simulink model "cubesatAttSim"  (R2024a)
settings: Solver=FixedStepAuto  StartTime=0.0  StopTime=7200  FixedStep=0.02  MaxStep=1  MinStep=0.001  RelTol=1e-3
model workspace (MAT data in the model file):
  earth_magnetic_field_body = [0 0 0]
  initial_angular_momentum_body = 0
  initial_position_iss_orbit = 0
  initial_quaterion_rotation = 0
  initial_velocity_iss_orbit = 0
  intertia_tensor = 0
  mass = 0
  maximum_sun_sensor_vision = 0
  reference_magnetic_field_direction = 0
  reference_sun_direction = 0
  wheel_distribution_matrix = [1  0  0  0; 0  1  0  0; 0  0  1  1]
libraries: aerolibutil x2, sharedtransform x1
settings Model: Creator=samuel  LastModifiedBy=joshu
settings OptimizationCC: ReuseModelBlockBuffer=off
settings DebuggingCC: AlgebraicLoopMsg=error  ArtificialAlgebraicLoopMsg=error
settings ModelReferenceCC: EnableRefExpFcnMdlSchedulingChecks=on
settings RTWCC: GPUComputeCapability=3.5

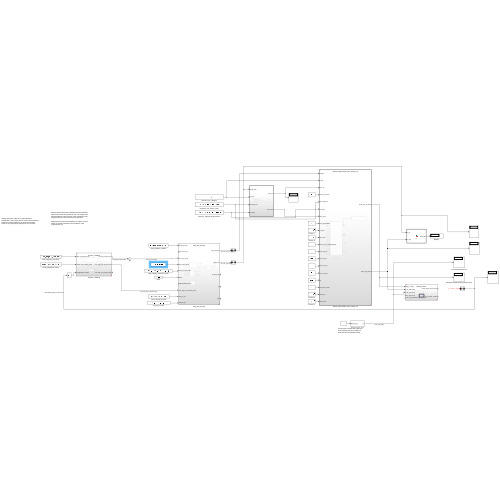
[thumbnail: Simulink's stored preview of the top-level diagram]
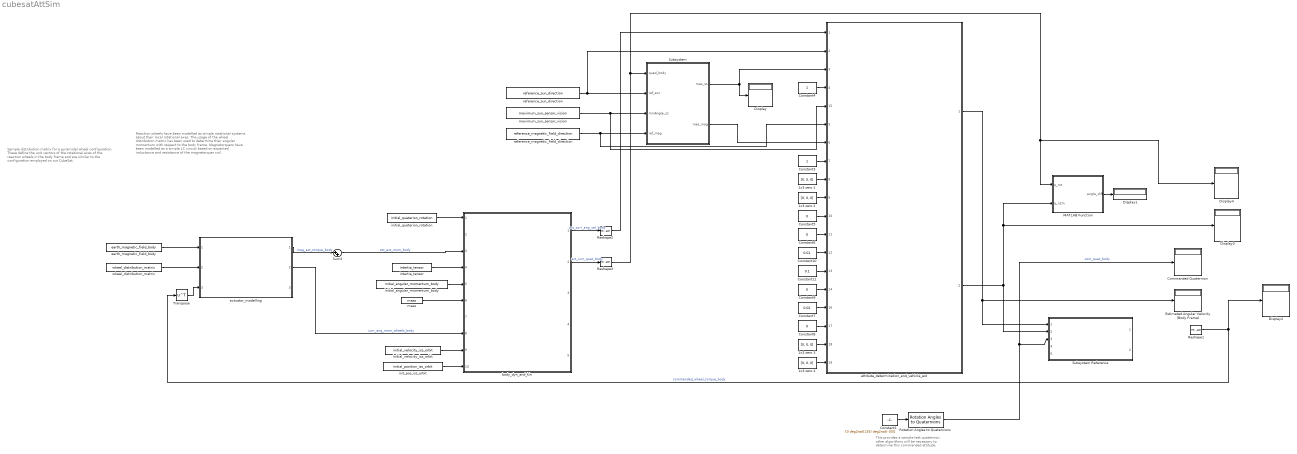
== system cubesatAttSim ==
  note: This provides a sample test quaternion, other algorithms will be necessary to determine this commanded attitude.
  note: Reaction wheels have been modelled as simple rotational systems about their local rotational axes. The usage of the wheel distribution matrix has been used to determine their angular momentum with respect to the body frame.
      |
      | Magnetorquers have been modelled as a simple LC circuit based on expected inductance and resistance of the magnetorquer coil.
  note: Sample distribution matrix for a pyramidal wheel configuration. These define the unit vectors of the rotational axes of the reaction wheels in the body frame and are similar to the configuration employed on our CubeSat.
  1x3 zero {1..4} (4 alike) : Constant  Value=[0, 0, 0]
  Commanded Quaternion : Display
  Constant1 : Constant  Value=[0 deg2rad(135) deg2rad(-30)]
  Constant10 : Constant  Value=0.01
  Constant11 : Constant  Value=0.1
  Constant3 : Constant  OutDataTypeStr=boolean
  Constant4 : Constant  OutDataTypeStr=boolean
  Constant5 : Constant  Value=0  OutDataTypeStr=boolean
  Constant6 : Constant  Value=0  OutDataTypeStr=boolean
  Constant7 : Constant  Value=0.02
  Constant8 : Constant  Value=0  OutDataTypeStr=boolean
  Constant9 : Constant  Value=0
  Display{,1..4} (5 alike) : Display
  Estimated Angular Velocity (Body Frame) : Display
  MATLAB Function : MATLAB Function  TreatAsAtomicUnit=on
  Reshape1 : Reshape  OutputDimensionality=Row vector (2-D)
  Reshape2 : Reshape  OutputDimensionality=Row vector (2-D)
  Reshape3 : Reshape  OutputDimensionality=Row vector (2-D)
  Rotation Angles to Quaternions : sharedtransform/Rotation Angles to Quaternions  rotationOrder=ZYX  aMode=aMode
  Subsystem : Subsystem  TreatAsAtomicUnit=on
  Subsystem Reference : Subsystem  ReferencedSubsystem=attitude_control
  Sum3 : Sum  Inputs=|++
  Transpose : Math  Operator=transpose
  actuator_modelling : Subsystem  ReferencedSubsystem=actuator_modelling
  attitude_determination_and_vehicle_est : Subsystem  TreatAsAtomicUnit=on  SystemSampleTime=0.02  ReferencedSubsystem=attitude_determination_and_vehicle_est
      settings: PortSchema="{\"entries\":[{\"content\":{\"sides\":[{\"content\":{\"connectorIds\":[\"In1\",\"In2\",\"In3\",\"In4\",\"In15\",\"In5\",\"In6\",\"In7\",\"In8\",\"In9\",\"In10\",\"In11\",\"In12\",\"In13\",\"In14\",\"In16\",\"In17\",\"In18\",\"In19\"]},\"type\":\"ConnectorPlacement.EquallySpacedRectSide\",\"uuid\":\"3b22937b-158d-42bc-8266-221df4d5bb4f\"},{\"content\":{\"connectorIds\":[\"Out1\",\"Out2\"],\"side\":\"RIGHT\"},\"type\":\"ConnectorPlacement.EquallySpacedRectSide\",\"uuid\":\"2d7976b0-5d09-4ece-a5b5-6f5d6f0d46dd\"},{\"content\":{\"side\":\"TOP\"},\"type\":\"ConnectorPlacement.EquallySpacedRectSide\",\"uuid\":\"411abe81-91ab-4e83-a0ca-8600290f09f5\"}]},\"type\":\"ConnectorPlacement.EquallySpacedConnector\",\"uuid\":\"dff24d4c-a30b-41c1-92cc-a12930c50369\"}],\"packageUris\":[\"http://schema.mathworks.com/mf0/Connector/R2020b\"],\"version\":\"1.0\"}"
  body_dyn_and_kin : Subsystem  ReferencedSubsystem=body_dyn_and_kin
  earth_magnetic_field_body : Constant  Value=earth_magnetic_field_body
  init_pos_iss_orbit : Constant  Value=initial_position_iss_orbit
  initial_angular_momentum_body : Constant  Value=initial_angular_momentum_body
  initial_quaterion_rotation : Constant  Value=initial_quaterion_rotation
  initial_velocity_iss_orbit : Constant  Value=initial_velocity_iss_orbit
  intertia_tensor : Constant  Value=intertia_tensor
  mass : Constant  Value=mass
  maximum_sun_sensor_vision : Constant  Value=maximum_sun_sensor_vision
  reference_magnetic_field_direction : Constant  Value=reference_magnetic_field_direction  VectorParams1D=off
  reference_sun_direction : Constant  Value=reference_sun_direction  VectorParams1D=off
  wheel_distribution_matrix : Constant  Value=wheel_distribution_matrix
  wires:
  intertia_tensor/1 -> body_dyn_and_kin/4
  wheel_distribution_matrix/1 -> actuator_modelling/2
  actuator_modelling/1 -> Sum3/1  "mag_act_torque_body"
  Sum3/1 -> body_dyn_and_kin/3  "tot_ext_mom_body"
  initial_angular_momentum_body/1 -> body_dyn_and_kin/5
  mass/1 -> body_dyn_and_kin/6
  actuator_modelling/2 -> body_dyn_and_kin/8  "curr_ang_mom_wheels_body"
  initial_velocity_iss_orbit/1 -> body_dyn_and_kin/9
  init_pos_iss_orbit/1 -> body_dyn_and_kin/10
  attitude_determination_and_vehicle_est/1 -> Subsystem Reference/1, Estimated Angular Velocity (Body Frame)/1
  attitude_determination_and_vehicle_est/2 -> Subsystem Reference/2, MATLAB Function/2(q_n2m), Display3/1
  Reshape1/1 -> Display2/1, Transpose/1  "commanded_wheel_torque_body"
  Transpose/1 -> actuator_modelling/3
  Constant1/1 -> Rotation Angles to Quaternions/1
  Rotation Angles to Quaternions/1 -> Subsystem Reference/3, Commanded Quaternion/1  "com_quat_body"
  earth_magnetic_field_body/1 -> actuator_modelling/1
  Subsystem/1(mes_ss) -> Display/1, attitude_determination_and_vehicle_est/3
  Subsystem/2(mes_mag) -> attitude_determination_and_vehicle_est/6
  Constant4/1 -> attitude_determination_and_vehicle_est/4
  1x3 zero 1/1 -> attitude_determination_and_vehicle_est/8
  1x3 zero 2/1 -> attitude_determination_and_vehicle_est/9
  Constant6/1 -> attitude_determination_and_vehicle_est/11
  Constant3/1 -> attitude_determination_and_vehicle_est/7
  Constant5/1 -> attitude_determination_and_vehicle_est/10
  Constant7/1 -> attitude_determination_and_vehicle_est/16
  Constant8/1 -> attitude_determination_and_vehicle_est/17
  Constant9/1 -> attitude_determination_and_vehicle_est/14
  Constant10/1 -> attitude_determination_and_vehicle_est/12
  Constant11/1 -> attitude_determination_and_vehicle_est/13
  1x3 zero 3/1 -> attitude_determination_and_vehicle_est/18
  1x3 zero 4/1 -> attitude_determination_and_vehicle_est/19
  maximum_sun_sensor_vision/1 -> attitude_determination_and_vehicle_est/15, Subsystem/3(minAngle_ss)
  reference_magnetic_field_direction/1 -> attitude_determination_and_vehicle_est/5, Subsystem/4(ref_mag)
  reference_sun_direction/1 -> attitude_determination_and_vehicle_est/2, Subsystem/2(ref_sun)
  MATLAB Function/1(angle_diff) -> Display1/1
  body_dyn_and_kin/2 -> Reshape3/1  "act_curr_quat_body"
  Reshape3/1 -> Subsystem/1(quad_body), Display4/1, MATLAB Function/1(q_rot)
  initial_quaterion_rotation/1 -> body_dyn_and_kin/1
  body_dyn_and_kin/1 -> Reshape2/1  "act_curr_ang_vel_body"
  Reshape2/1 -> attitude_determination_and_vehicle_est/1
  ? -> Reshape1/1

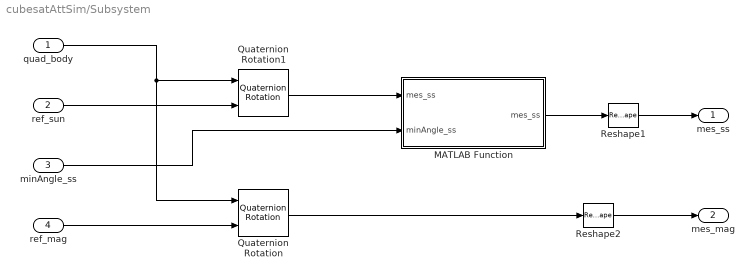
== system cubesatAttSim/Subsystem ==
  quad_body : Inport
  ref_sun : Inport  Port=2
  minAngle_ss : Inport  Port=3
  ref_mag : Inport  Port=4
  MATLAB Function : MATLAB Function  TreatAsAtomicUnit=on
  Quaternion Rotation : aerolibutil/Quaternion Rotation
  Quaternion Rotation1 : aerolibutil/Quaternion Rotation
  Reshape1 : Reshape  OutputDimensionality=Row vector (2-D)
  Reshape2 : Reshape  OutputDimensionality=Row vector (2-D)
  mes_ss : Outport
  mes_mag : Outport  Port=2
  wires:
  ref_mag/1 -> Quaternion Rotation/2
  quad_body/1 -> Quaternion Rotation1/1, Quaternion Rotation/1
  ref_sun/1 -> Quaternion Rotation1/2
  Quaternion Rotation1/1 -> MATLAB Function/1("mes_ss ")
  minAngle_ss/1 -> MATLAB Function/2(minAngle_ss)
  MATLAB Function/1(mes_ss) -> Reshape1/1
  Quaternion Rotation/1 -> Reshape2/1
  Reshape1/1 -> mes_ss/1
  Reshape2/1 -> mes_mag/1

== matlab function cubesatAttSim/MATLAB Function ==
  data: q_rot input; angle_diff output; q_n2m input
function angle_diff = fcn(q_rot,q_n2m)

    q_rel = quatmultiply(q_rot, quatinv(q_n2m));
    cos_theta_over_2 = abs(q_rel(1));
    angle_diff = 2 * acos(cos_theta_over_2)*180/pi;

== matlab function cubesatAttSim/Subsystem/MATLAB Function ==
  data: mes_ss input; mes_ss output; minAngle_ss input
function mes_ss = fcn(mes_ss, minAngle_ss)
    mes_ss = (abs(mes_ss) > cosd(minAngle_ss)).*mes_ss;
